simulink model "OAR"  (R2019a)
settings: Solver=FixedStepAuto  StartTime=0.0  StopTime=inf  RelTol=1e-3  EnableMultiTasking=on
libraries: arduinolib x4, simulink x2, LCDlib x1, arduinosensorlib x1
settings Model: SimulationMode=external  ExtModeTrigDuration=2  Creator=rishi  LastModifiedBy=rishi
settings OptimizationCC: EnhancedBackFolding=on  PassReuseOutputArgsAs=Individual arguments  MaxStackSize=64  OptimizeBlockOrder=speed  DifferentSizesBufferReuse=on  OptimizationCustomize=off
settings DebuggingCC: ParameterTunabilityLossMsg=error
settings HardwareCC: ProdBitPerInt=16  ProdBitPerPointer=16  ProdBitPerSizeT=16  ProdBitPerPtrDiffT=16  ProdLargestAtomicFloat=None  ProdWordSize=8  ProdHWDeviceType=Atmel->AVR
settings SFSimCC: MATLABDynamicMemAlloc=off
settings RTWCC: SystemTargetFile=ert.tlc  HardwareBoard=Arduino Uno  TLCOptions=-aInlineSetEventsForThisBaseRateFcn=TLC_FALSE -aSuppressMultiTaskScheduler=TLC_FALSE -aRateBasedStepFcn=1  TemplateMakefile=ert_default_tmf  GenerateReport=on  Toolchain=Arduino AVR  BuildConfiguration=Faster Runs  IncludeHyperlinkInReport=on  LaunchReport=on  GenerateTraceInfo=on  GenerateTraceReport=on  GenerateTraceReportSl=on  GenerateTraceReportSf=on  GenerateTraceReportEml=on
settings CodeAppCC: ForceParamTrailComments=on  IgnoreCustomStorageClasses=off  OperatorAnnotations=on  SimulinkDataObjDesc=on  SFDataObjDesc=on  InsertBlockDesc=on
settings ERTTargetCC: SupportContinuousTime=on  SupportVariableSizeSignals=on  ExtModeStaticAllocSize=250

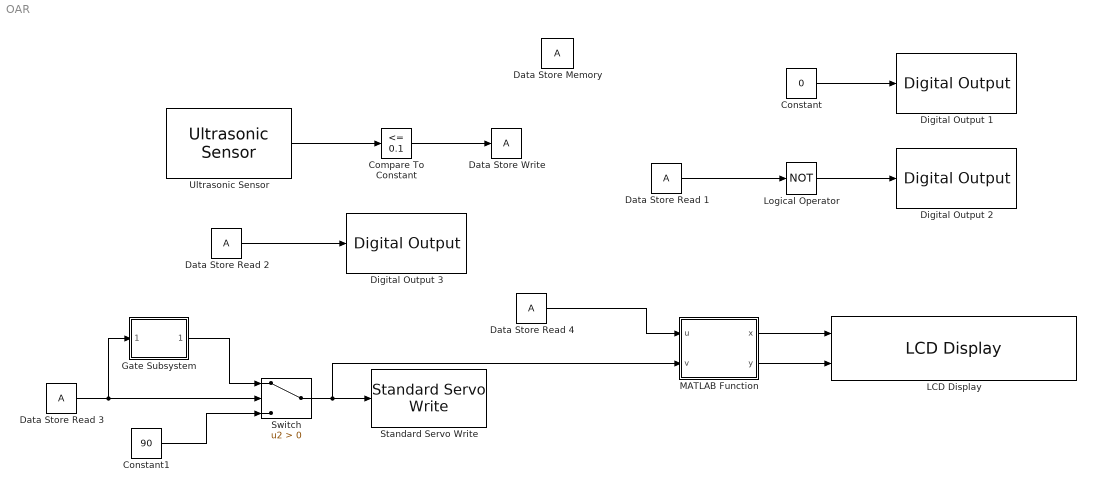
== system OAR ==
  Compare To Constant : simulink/Logic and Bit Operations/Compare To Constant  relop=<=  const=0.1  OutDataTypeStr=boolean
  Constant : Constant  Value=0
  Constant1 : Constant  Value=90
  Data Store Memory : DataStoreMemory  ReadBeforeWriteMsg=warning  WriteAfterWriteMsg=warning  WriteAfterReadMsg=warning  ShowAdditionalParam=off
  Data Store Read {1..4} (4 alike) : DataStoreRead
  Data Store Write : DataStoreWrite
  Digital Output 1 : arduinolib/Digital Output  pinNumber=6  blockPlatform=arduino
  Digital Output 2 : arduinolib/Digital Output  pinNumber=5  blockPlatform=arduino
  Digital Output 3 : arduinolib/Digital Output  pinNumber=4  blockPlatform=arduino
  Gate Subsystem : Subsystem
  LCD Display : LCDlib/LCD Display  pins=[3, 2, 10, 11, 12, 13]
      settings: SourceProductName=LCD Library
  Logical Operator : Logic  Operator=NOT  AllPortsSameDT=off  OutDataTypeStr=boolean
  MATLAB Function : MATLAB Function  TreatAsAtomicUnit=on
  Standard Servo Write : arduinolib/Standard Servo Write  pinNumber=9  ServoIndex=0  blockPlatform=ARDUINO
      settings: SourceProductName=Simulink Support Package for Arduino Hardware
  Switch : Switch  Criteria=u2 > Threshold
  Ultrasonic Sensor : arduinosensorlib/Ultrasonic Sensor  NumSignalPins=2  TrigPin=7  EchoPin=8  SignalPin=3  SampleTime_=1  blockPlatform=ARDUINO
      settings: SourceProductName=Simulink Support Package for Arduino Hardware  SourceProductBaseCode=ARDUINO
  wires:
  Logical Operator/1 -> Digital Output 2/1
  Ultrasonic Sensor/1 -> Compare To Constant/1
  Compare To Constant/1 -> Data Store Write/1
  Data Store Read 1/1 -> Logical Operator/1
  Constant/1 -> Digital Output 1/1
  Data Store Read 2/1 -> Digital Output 3/1
  Data Store Read 3/1 -> Gate Subsystem/1(Input), Switch/2
  Constant1/1 -> Switch/3
  Gate Subsystem/1(Out 1) -> Switch/1
  MATLAB Function/2(y) -> LCD Display/2
  MATLAB Function/1(x) -> LCD Display/1
  Switch/1 -> MATLAB Function/2(v), Standard Servo Write/1
  Data Store Read 4/1 -> MATLAB Function/1(u)

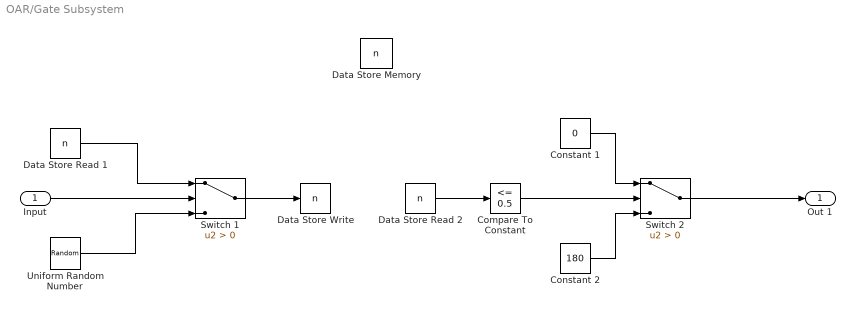
== system OAR/Gate Subsystem ==
  Input : Inport
  Compare To Constant : simulink/Logic and Bit Operations/Compare To Constant  relop=<=  const=0.5  OutDataTypeStr=boolean
  Constant 1 : Constant  Value=0
  Constant 2 : Constant  Value=180
  Data Store Memory : DataStoreMemory  DataStoreName=n  ReadBeforeWriteMsg=warning  WriteAfterWriteMsg=warning  WriteAfterReadMsg=warning  ShowAdditionalParam=off  OutDataTypeStr=double
      settings: LockScale=on
  Data Store Read 1 : DataStoreRead  DataStoreName=n
  Data Store Read 2 : DataStoreRead  DataStoreName=n
  Data Store Write : DataStoreWrite  DataStoreName=n
  Switch 1 : Switch  Criteria=u2 > Threshold
  Switch 2 : Switch  Criteria=u2 > Threshold
  Uniform Random Number : UniformRandomNumber  Minimum=0  SampleTime=1
  Out 1 : Outport
  wires:
  Compare To Constant/1 -> Switch 2/2
  Switch 2/1 -> Out 1/1
  Constant 2/1 -> Switch 2/3
  Constant 1/1 -> Switch 2/1
  Input/1 -> Switch 1/2
  Uniform Random Number/1 -> Switch 1/3
  Data Store Read 1/1 -> Switch 1/1
  Switch 1/1 -> Data Store Write/1
  Data Store Read 2/1 -> Compare To Constant/1

== matlab function OAR/MATLAB Function ==
  data: x output; u input; y output; v input
function [x,y] = fcn(u,v)
if u==0
    x = [68 67 32 109 111 116 111 114 32 82 80 77 58 32 32 32];
    y = [51 48 48 32 32 32 32 32 32 32 32 32 32 32 32 32];
else
    x = [65 108 101 114 116 33 32 32 32 32 32 32 32 32 32 32];
    if v==0
        y = [84 117 114 110 105 110 103 32 82 105 103 104 105 32 32 32];
    else
        y = [84 117 114 110 105 110 103 32 76 101 102 116 32 32 32 32];
    end
end
